simulink model "System_Model"  (R2017b)
settings: Solver=VariableStepAuto  StartTime=0.0  StopTime=10.0  RelTol=1e-3
values from neighbouring files (symbols this model uses):
  A = [-a 0 -b ... (first row only)    [Initialize_Parameters.m]    (also in Initialize_Parameters_MATLAB_Functions.m)
  B = [c ... (first row only)    [Initialize_Parameters.m]    (also in Initialize_Parameters_MATLAB_Functions.m)
settings Model: Creator=pawestlu  LastModifiedBy=pawestlu

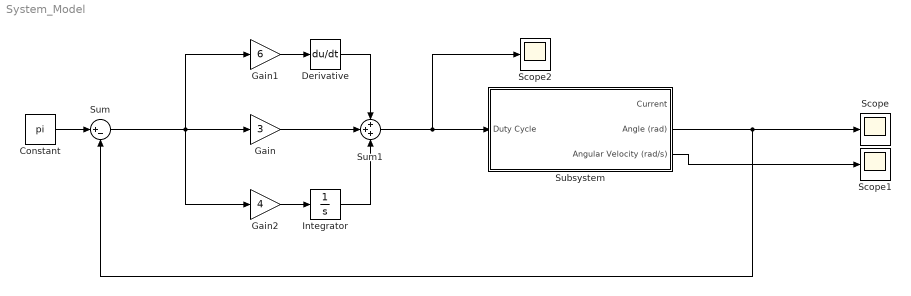
== system System_Model ==
  Constant : Constant  Value=pi
  Derivative : Derivative
  Gain : Gain  Gain=3
  Gain1 : Gain  Gain=6
  Gain2 : Gain  Gain=4
  Integrator : Integrator
  Scope : Scope
  Scope1 : Scope
  Scope2 : Scope
  Subsystem : Subsystem
  Sum : Sum  Inputs=|+-
  Sum1 : Sum  Inputs=+++
  wires:
  Subsystem/2(Angle (rad)) -> Sum/2, Scope/1
  Subsystem/3(Angular Velocity (rad/s)) -> Scope1/1
  Sum/1 -> Gain2/1, Gain1/1, Gain/1
  Constant/1 -> Sum/1
  Sum1/1 -> Scope2/1, Subsystem/1(Duty Cycle)
  Gain1/1 -> Derivative/1
  Gain/1 -> Sum1/2
  Derivative/1 -> Sum1/1
  Integrator/1 -> Sum1/3
  Gain2/1 -> Integrator/1

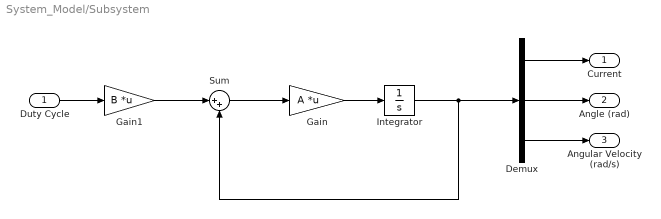
== system System_Model/Subsystem ==
  Duty Cycle : Inport
  Demux : Demux  Outputs=3
  Gain : Gain  Gain=A  Multiplication=Matrix(K*u)
  Gain1 : Gain  Gain=B  Multiplication=Matrix(K*u)
  Integrator : Integrator
  Sum : Sum  Inputs=|++
  Current : Outport
  Angle (rad) : Outport  Port=2
  Angular Velocity (rad/s) : Outport  Port=3
  wires:
  Sum/1 -> Gain/1
  Gain1/1 -> Sum/1
  Demux/2 -> Angle (rad)/1
  Gain/1 -> Integrator/1
  Integrator/1 -> Demux/1, Sum/2
  Duty Cycle/1 -> Gain1/1
  Demux/1 -> Current/1
  Demux/3 -> Angular Velocity (rad/s)/1
